simulink model "BLDC_Motor_FOC_rev6"  (R2017b)
settings: Solver=FixedStepDiscrete  StartTime=0.0  StopTime=2  MaxStep=1e-4  RelTol=1e-4
libraries: powerlib x11, powerlib_meascontrol x1
settings Model: Creator=Nick  LastModifiedBy=Nick
settings CodeAppCC: StateflowObjectComments=on

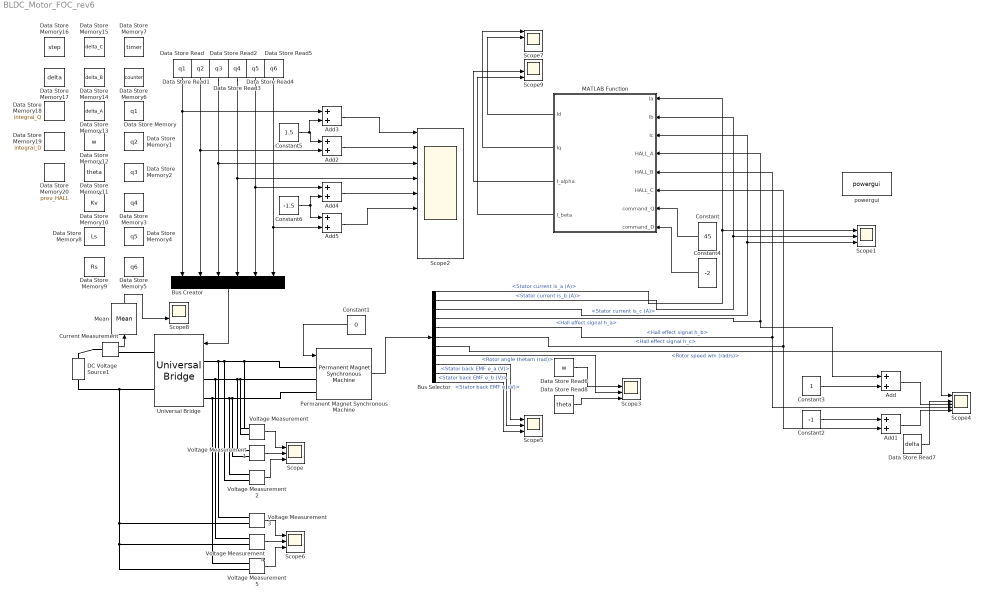
== system BLDC_Motor_FOC_rev6 ==
  Add{,1..5} (6 alike) : Sum
  Bus Creator : BusCreator  Inputs=6
  Bus Selector : BusSelector  OutputSignals=Stator current is_a (A),Stator current is_b (A),Stator current is_c (A),Hall effect signal h_a,Hall effect signal h_b,Hall effect signal h_c,Rotor speed wm (rad/s),Rotor angle thetam (rad),Stator back EMF e_a (V),Stator back EMF e_b (V),Stator back EMF e_cV)
  Constant : Constant  Value=45
  Constant1 : Constant  Value=0
  Constant2 : Constant  Value=-1
  Constant3 : Constant
  Constant4 : Constant  Value=-2
  Constant5 : Constant  Value=1.5
  Constant6 : Constant  Value=-1.5
  Current Measurement : powerlib/Measurements/Current Measurement  PhasorSimulation=off  OutputType=Complex  PSBequivalent=0
  DC Voltage Source1 : powerlib/Electrical Sources/DC Voltage Source  Amplitude=48  Measurements=None
  Data Store Memory : DataStoreMemory  DataStoreName=q1  ReadBeforeWriteMsg=warning  WriteAfterWriteMsg=warning  WriteAfterReadMsg=warning  ShowAdditionalParam=off  OutDataTypeStr=double
  Data Store Memory1 : DataStoreMemory  DataStoreName=q2  ReadBeforeWriteMsg=warning  WriteAfterWriteMsg=warning  WriteAfterReadMsg=warning  ShowAdditionalParam=off  OutDataTypeStr=double
  Data Store Memory10 : DataStoreMemory  DataStoreName=Kv  ReadBeforeWriteMsg=warning  WriteAfterWriteMsg=warning  WriteAfterReadMsg=warning  InitialValue=100  ShowAdditionalParam=off  OutDataTypeStr=double
  Data Store Memory11 : DataStoreMemory  DataStoreName=theta  ReadBeforeWriteMsg=warning  WriteAfterWriteMsg=warning  WriteAfterReadMsg=warning  ShowAdditionalParam=off  OutDataTypeStr=double
  Data Store Memory12 : DataStoreMemory  DataStoreName=w  ReadBeforeWriteMsg=warning  WriteAfterWriteMsg=warning  WriteAfterReadMsg=warning  ShowAdditionalParam=off  OutDataTypeStr=double
  Data Store Memory13 : DataStoreMemory  DataStoreName=delta_A  ReadBeforeWriteMsg=warning  WriteAfterWriteMsg=warning  WriteAfterReadMsg=warning  ShowAdditionalParam=off  OutDataTypeStr=double
  Data Store Memory14 : DataStoreMemory  DataStoreName=delta_B  ReadBeforeWriteMsg=warning  WriteAfterWriteMsg=warning  WriteAfterReadMsg=warning  ShowAdditionalParam=off  OutDataTypeStr=double
  Data Store Memory15 : DataStoreMemory  DataStoreName=delta_C  ReadBeforeWriteMsg=warning  WriteAfterWriteMsg=warning  WriteAfterReadMsg=warning  ShowAdditionalParam=off  OutDataTypeStr=double
  Data Store Memory16 : DataStoreMemory  DataStoreName=step  ReadBeforeWriteMsg=warning  WriteAfterWriteMsg=warning  WriteAfterReadMsg=warning  InitialValue=5e-6  ShowAdditionalParam=off  OutDataTypeStr=double
  Data Store Memory17 : DataStoreMemory  DataStoreName=delta  ReadBeforeWriteMsg=warning  WriteAfterWriteMsg=warning  WriteAfterReadMsg=warning  ShowAdditionalParam=off  OutDataTypeStr=double
  Data Store Memory18 : DataStoreMemory  DataStoreName=integral_Q  ReadBeforeWriteMsg=warning  WriteAfterWriteMsg=warning  WriteAfterReadMsg=warning  ShowAdditionalParam=off  OutDataTypeStr=double
  Data Store Memory19 : DataStoreMemory  DataStoreName=integral_D  ReadBeforeWriteMsg=warning  WriteAfterWriteMsg=warning  WriteAfterReadMsg=warning  ShowAdditionalParam=off  OutDataTypeStr=double
  Data Store Memory2 : DataStoreMemory  DataStoreName=q3  ReadBeforeWriteMsg=warning  WriteAfterWriteMsg=warning  WriteAfterReadMsg=warning  ShowAdditionalParam=off  OutDataTypeStr=double
  Data Store Memory20 : DataStoreMemory  DataStoreName=prev_HALL  ReadBeforeWriteMsg=warning  WriteAfterWriteMsg=warning  WriteAfterReadMsg=warning  ShowAdditionalParam=off  OutDataTypeStr=double
  Data Store Memory3 : DataStoreMemory  DataStoreName=q4  ReadBeforeWriteMsg=warning  WriteAfterWriteMsg=warning  WriteAfterReadMsg=warning  ShowAdditionalParam=off  OutDataTypeStr=double
  Data Store Memory4 : DataStoreMemory  DataStoreName=q5  ReadBeforeWriteMsg=warning  WriteAfterWriteMsg=warning  WriteAfterReadMsg=warning  ShowAdditionalParam=off  OutDataTypeStr=double
  Data Store Memory5 : DataStoreMemory  DataStoreName=q6  ReadBeforeWriteMsg=warning  WriteAfterWriteMsg=warning  WriteAfterReadMsg=warning  ShowAdditionalParam=off  OutDataTypeStr=double
  Data Store Memory6 : DataStoreMemory  DataStoreName=counter  ReadBeforeWriteMsg=warning  WriteAfterWriteMsg=warning  WriteAfterReadMsg=warning  ShowAdditionalParam=off  OutDataTypeStr=double
  Data Store Memory7 : DataStoreMemory  DataStoreName=timer  ReadBeforeWriteMsg=warning  WriteAfterWriteMsg=warning  WriteAfterReadMsg=warning  ShowAdditionalParam=off  OutDataTypeStr=double
  Data Store Memory8 : DataStoreMemory  DataStoreName=Ls  ReadBeforeWriteMsg=warning  WriteAfterWriteMsg=warning  WriteAfterReadMsg=warning  InitialValue=.0085  ShowAdditionalParam=off  OutDataTypeStr=double
  Data Store Memory9 : DataStoreMemory  DataStoreName=Rs  ReadBeforeWriteMsg=warning  WriteAfterWriteMsg=warning  WriteAfterReadMsg=warning  InitialValue=.0485  ShowAdditionalParam=off  OutDataTypeStr=double
  Data Store Read : DataStoreRead  DataStoreName=q1
  Data Store Read1 : DataStoreRead  DataStoreName=q2
  Data Store Read2 : DataStoreRead  DataStoreName=q3
  Data Store Read3 : DataStoreRead  DataStoreName=q4
  Data Store Read4 : DataStoreRead  DataStoreName=q5
  Data Store Read5 : DataStoreRead  DataStoreName=q6
  Data Store Read6 : DataStoreRead  DataStoreName=w
  Data Store Read7 : DataStoreRead  DataStoreName=delta
  Data Store Read8 : DataStoreRead  DataStoreName=theta
  MATLAB Function : MATLAB Function  TreatAsAtomicUnit=on
  Mean : powerlib_meascontrol/Measurements/Mean  Freq=60  Vinit=0  Ts=5e-05
  Permanent Magnet Synchronous Machine : powerlib/Machines/Permanent Magnet Synchronous Machine  NbPhases=3  FluxDistribution=Trapezoidal  RotorType=Round  MechanicalLoad=Torque Tm  PresetModel=No  ShowDetailedParameters=on  MeasurementBus=off  Resistance=0.0485  Inductance=8.5e-3  dqInductances=[8.5e-3,8.5e-3]  La=0.000395  MachineConstant=Voltage Constant (V_peak L-L / krpm)  Flux=0.1194  VoltageCst=100.0283  TorqueCst=0.9552  Flat=120  Mechanical=[0.0027 0.0004924 4 0]  PolePairs=4  InitialConditions=[0,0, 0,0]  InitialConditions5ph=[0 0 0 0 0 0]  TsPowergui=0  TsBlock=-1  RefAngle=Aligned with phase A axis (original Park)
      settings: SourceProductName=Simscape Power Systems
  Scope{,1,5..6,8} (5 alike) : Scope  NumInputPorts=3
  Scope2 : Scope  NumInputPorts=9
  Scope3 : Scope  NumInputPorts=4
  Scope4 : Scope  NumInputPorts=6
  Scope7 : Scope  NumInputPorts=4
  Scope9 : Scope  NumInputPorts=6
  Universal Bridge : powerlib/Power Electronics/Universal Bridge  Arms=3  SnubberResistance=1e5  SnubberCapacitance=inf  Device=MOSFET / Diodes  Ron=1e-3  Lon=0  ForwardVoltages="[  0  0  ]"  ForwardVoltage=0  GTOparameters=[ 10e-6 , 20e-6 ]  IGBTparameters=[ 1e-6 , 2e-6 ]  Measurements=None  Measurements_2=None  converterType=Rectifier
  Voltage Measurement{,1..5} (6 alike) : powerlib/Measurements/Voltage Measurement  PhasorSimulation=off  OutputType=Complex  PSBequivalent=0
  powergui : powerlib/powergui  Priority=1  SimulationMode=Discrete  SampleTime=5e-5  frequency=60  Iterations=50  frequencyindice=0  Pbase=100e6  ErrMax=1e-4  UnitsV=kV  UnitsW=MW  buscounter=0  FunctionMessages=off  echomessages=off  EnableUseOfTLC=off  CurrentSourceSwitches=off  DisableSnubberDevices=off  DisableRonSwitches=off  DisableVfSwitches=off  DisplayEquations=off  SolverType=Tustin/Backward Euler (TBE)  Interpol=off  ExternalGateDelay=off  methode=off  Ts=100  x0status=blocks  SPID=off  SwTol=0  HookPort=off  RestoreLinks=warning  ResistiveCurrentMeasurement=off  Frange=[0:2:500]  Ylog=off  Xlog=on  ShowGrid=off  save=off  variable=ZData  structure=0  ZoomFFT=off  StartTime=0.0  cycles=1  DisplayStyle=1  fundamental=60  FreqAxis=off  MaxFrequency=1000  frequencyindicesteady=1  RmsSteady=1  display=off
  wires:
  Permanent Magnet Synchronous Machine/1 -> Bus Selector/1
  Bus Selector/1 -> MATLAB Function/1(Ia), Scope1/1  "<Stator current is_a (A)>"
  Constant/1 -> MATLAB Function/7(command_Q)
  Bus Selector/5 -> Scope4/5, MATLAB Function/5(HALL_B)  "<Hall effect signal h_b>"
  Bus Selector/6 -> Add1/2, MATLAB Function/6(HALL_C)  "<Hall effect signal h_c>"
  Bus Selector/4 -> Add/1, MATLAB Function/4(HALL_A)  "<Hall effect signal h_a>"
  Voltage Measurement/1 -> Scope/1
  Bus Creator/1 -> Universal Bridge/1
  Constant3/1 -> Add/2
  Constant2/1 -> Add1/1
  Add1/1 -> Scope4/6
  Add/1 -> Scope4/4
  Data Store Read/1 -> Add3/1, Bus Creator/1
  Data Store Read2/1 -> Scope2/3, Bus Creator/3
  Data Store Read3/1 -> Scope2/4, Bus Creator/4
  Data Store Read4/1 -> Add4/1, Bus Creator/5
  Constant1/1 -> Permanent Magnet Synchronous Machine/1
  Bus Selector/7 -> Scope4/1  "<Rotor speed wm (rad/s)>"
  Voltage Measurement4/1 -> Scope6/2
  Voltage Measurement5/1 -> Scope6/3
  Data Store Read1/1 -> Add2/2, Bus Creator/2
  Bus Selector/8 -> Scope3/3  "<Rotor angle thetam (rad)>"
  Add2/1 -> Scope2/2
  Constant5/1 -> Add3/2, Add2/1
  Add4/1 -> Scope2/5
  Add5/1 -> Scope2/6
  Constant6/1 -> Add5/1, Add4/2
  Data Store Read5/1 -> Add5/2, Bus Creator/6
  Bus Selector/9 -> Scope5/1  "<Stator back EMF e_a (V)>"
  Bus Selector/10 -> Scope5/2  "<Stator back EMF e_b (V)>"
  Bus Selector/11 -> Scope5/3  "<Stator back EMF e_cV)>"
  Add3/1 -> Scope2/1
  Voltage Measurement3/1 -> Scope6/1
  Bus Selector/2 -> MATLAB Function/2(Ib), Scope1/2  "<Stator current is_b (A)>"
  Bus Selector/3 -> MATLAB Function/3(Ic), Scope1/3  "<Stator current is_c (A)>"
  Voltage Measurement1/1 -> Scope/2
  Voltage Measurement2/1 -> Scope/3
  Data Store Read6/1 -> Scope3/2
  Data Store Read7/1 -> Scope4/3
  MATLAB Function/1(Id) -> Scope7/2
  MATLAB Function/2(Iq) -> Scope7/1
  Data Store Read8/1 -> Scope3/4
  Constant4/1 -> MATLAB Function/8(command_D)
  Current Measurement/1 -> Mean/1
  Mean/1 -> Scope8/3
  MATLAB Function/3(I_alpha) -> Scope9/4
  MATLAB Function/4(I_beta) -> Scope9/6
  connections:
  Universal Bridge/LConn1 -- Voltage Measurement3/LConn1 -- Voltage Measurement2/LConn2 -- Voltage Measurement/LConn1 -- Permanent Magnet Synchronous Machine/LConn1
  Universal Bridge/LConn2 -- Voltage Measurement4/LConn1 -- Voltage Measurement1/LConn1 -- Permanent Magnet Synchronous Machine/LConn2 -- Voltage Measurement/LConn2
  Universal Bridge/LConn3 -- Voltage Measurement5/LConn1 -- Voltage Measurement2/LConn1 -- Permanent Magnet Synchronous Machine/LConn3 -- Voltage Measurement1/LConn2
  Universal Bridge/RConn2 -- Voltage Measurement3/LConn2 -- Voltage Measurement4/LConn2 -- Voltage Measurement5/LConn2 -- DC Voltage Source1/LConn1
  Universal Bridge/RConn1 -- Current Measurement/RConn1
  Current Measurement/LConn1 -- DC Voltage Source1/RConn1

== matlab function BLDC_Motor_FOC_rev6/MATLAB Function ==
  settings: updateMethod=DISCRETE  sampleTime=50e-7  description=Direct Current calculated from the parke transformation
  data Id settings: description=Direct Current calcultated from parke transformation
  data Iq settings: description=Quadrature Current calcultated from parke transformation
  data Ia settings: description=Phase A Armature current from motor
  data Ib settings: description=Phase B Armature current from motor
  data Ic settings: description=Phase C Armature current from motor
  data HALL_A settings: description=Input from hall affect sensor Phase A
  data HALL_B settings: description=Input from hall affect sensor Phase B
  data HALL_C settings: description=Input from hall affect sensor Phase C
  data command_Q settings: description=Input command from user, a percentage of 0 to 30 amps.
  data q1 settings: description=Gate of q1 (Top FET of Phase A)
  data q2 settings: description=Gate of q2 (Bottom FET of Phase A)
  data q3 settings: description=Gate of q3 (Top FET of Phase B)
  data q4 settings: description=Gate of q4 (Bottom FET of Phase B)
  data q5 settings: description=Gate of q5 (Top FET of Phase C)
  data q6 settings: description=Gate of q6 (Bottom FET of Phase C)
  data counter settings: description=Counter variable used to help set PWM in Trapezoid control mode
  data timer settings: description=Keeps a running time of the program
  data I_alpha settings: description=Corrected Phase A current after PI controller and Parke/Clarke transforms
  data I_beta settings: description=Corrected Phase B current after PI controller and Parke/Clarke transforms
  data theta settings: description=Position of the motor calcultated using time and HALL effect sensors
  data Kv settings: description=Unused variable at the moment
  data w settings: description=Speed of the motor calcultated using time and HALL effect sensors
  data delta_A settings: description=Value of HALL effect sensor A from previous step
  data delta_B settings: description=Value of HALL effect sensor B from previous step
  data delta_C settings: description=Value of HALL effect sensor C from previous step
  data step settings: description=Length of individual time step
  data delta settings: description=Holds the time since the last HALL effect sensor changed
  data integral_Q settings: description=Running value of the integral of the Quadrature current by the PI controller
  data integral_D settings: description=Running value of the integral of the Direct current by the PI controller
  data prev_HALL settings: description=Describes which HALL effect sensor was the last to change to determine the direction of the motor
  data: Id output; Iq output; Ia input size=1; Ib input size=1; Ic input size=1; HALL_A input; HALL_B input; HALL_C input size=1; command_Q input size=1; q1 data_store_memory; q2 data_store_memory; q3 data_store_memory; q4 data_store_memory; q5 data_store_memory; q6 data_store_memory; counter data_store_memory; timer data_store_memory; I_alpha output; I_beta output; theta data_store_memory; Kv data_store_memory; w data_store_memory; delta_A data_store_memory; delta_B data_store_memory; delta_C data_store_memory; step data_store_memory; delta data_store_memory; integral_Q data_store_memory; integral_D data_store_memory; prev_HALL data_store_memory; command_D input
function [Id,Iq,I_alpha, I_beta] = control(Ia,Ib,Ic,HALL_A,HALL_B,HALL_C,command_Q,command_D)

% most of the global variables that are used throughout the program are
% created and listed here
global counter     % Counter for duty cycle
global delta       % Time since previous HALL sensor
global step        % Sample period
global delta_A     % Value of HALL A one step prior
global delta_B     % Value of HALL B one step prior
global delta_C     % Value of HALL C one step prior
global w           % Speed in radians per second
global theta       % Angle in radians
global timer       % Time since start of program
global integral_Q  % Value of descrete integral for Q current
global integral_D  % Value of descrete integral for D current

A = 0; % Sets initial value for phase A voltage
B = 0; % Sets initial value for phase B voltage
C = 0; % Sets initial value for phase C voltage

% Using current readings from the current sensors we calculate the alpha
% and beta currents of the motor
[I_alpha,I_beta] = clarke(Ia,Ib,Ic);

% Continuously tracking the amount of time since the previous Hall effecto
% sensor reading to keep track of speed and position of motor
delta = delta + step; 

% Continuously keeps track of the time passed since the beginning of the
% program to change when we switch from trapezpoidal to FOC
timer = timer + step; 

if timer >= 0.0001 % Problem in function fix later
    read_pos(HALL_A,HALL_B,HALL_C); % Keeps track of the position of the motor
end


delta_A = HALL_A; % Saves previous state of Hall effect sensor A
delta_B = HALL_B; % Saves previous state of Hall effect sensor B
delta_C = HALL_C; % Saves previous state of Hall effect sensor C

theta = theta + w*step; % Integrating to keep track of angle

[Id,Iq] = park(I_alpha,I_beta,4*theta); % Calculate direct and quadrature currents

counter = counter + 1; % Keeping track of duty cycle

% Runs trapezoidal control for .1 seconds then flips to FOC
if timer < .1
    trapezoid(command_Q,HALL_A,HALL_B,HALL_C);

% Flipping Field Oriented Control
else
    % PI control for quadrature current
    error_Q = ((command_Q/100)*30) - Iq;
    integral_Q = integral_Q + (error_Q*step);
    u_Q = 1000*integral_Q + 1000*error_Q;
    
    % PI control for direct current
    error_D = (command_D - Id);
    integral_D = integral_D + (error_D*step);
    u_D = 1000*integral_D + 1000*error_D;
    
    % Calculate inverse parke transformation for PI control output
    [I_alpha,I_beta] = inverse_parke(u_D,u_Q,4*theta);
    
    % Calculate inverse clarke transformation for PI control output
    [A,B,C] = inverse_clarke(I_alpha,I_beta);
    % Raises or lowers voltages based on coontrol signal
    regulate(A,B,C,Ia,Ib,Ic); 
end
    
end

% regulate is a function that comapares the values of the 
% voltages on the line and tries to raise them if they are below
% the value that the PI controller is asking for
% or lowers them if the actual value is less than what the PI controller
% asks for
function regulate(command_A,command_B,command_C,A,B,C)
    global q1
    global q2
    global q3
    global q4
    global q5
    global q6
    
    if A < command_A
        q1 = 1;
        q2 = 0;
    else
        q1 = 0;
        q2 = 1;
    end
    if B < command_B
        q3 = 1;
        q4 = 0;
    else
        q3 = 0;
        q4 = 1;
    end
    if C < command_C
        q5 = 1;
        q6 = 0;
    else
        q5 = 0;
        q6 = 1;
    end
end


% This function takes in alpha/beta voltages/currents and the angle of the
% motor computes the direct/quadrature voltages/currents
function [d,q] = park(alpha,beta,theta)
    d = cos(theta)*alpha + sin(theta)*beta;
    q = cos(theta)*beta - sin(theta)*alpha;
end

% This function takes in a/b/c voltages/currents
% and computes the alpha/beta voltages/currents
function [alpha,beta] = clarke(a,b,c)
    alpha = a;
    beta = (1/(sqrt(3))*(b-c));
end

% This function takes in direct/gaudrature voltages/currents
% and the angle of the motor and performs the reverse parke transformation
% giving alpha/beta voltages/currents
function [alpha,beta] = inverse_parke(d,q,theta)
    alpha = d*cos(theta) - q*sin(theta);
    beta = q*cos(theta) + d*sin(theta);
end


% This function takes in alpha/beta voltages/currents and 
% performs the reverse clarke transformation and returns a/b/c
% voltages/currents
function [a,b,c] = inverse_clarke(alpha,beta)
    a = alpha;
    b = (1/2)*((-alpha) + (sqrt(3)*beta));
    c = (1/2)*((-alpha) - (sqrt(3)*beta));
end

% This function takes in a counter which helps define a duty cycle
% along with a command 0 to 100 percent and the position of the motor
% via the hall affect sensors and produces a trapazoid output signal
% to the 3 half bridges
function trapezoid(command,HALL_A,HALL_B,HALL_C)
    global q1
    global q2
    global q3
    global q4
    global q5
    global q6
    global counter
    if counter <= command
        if HALL_A && ~HALL_B && HALL_C
            q1 = 1;
            q2 = 0;
            q3 = 0;
            q4 = 1;
            q5 = 1;
            q6 = 0;

        elseif HALL_A && ~HALL_B && ~HALL_C
            q1 = 1;
            q2 = 0;
            q3 = 0;
            q4 = 1;
            q5 = 0;
            q6 = 1;

        elseif HALL_A && HALL_B && ~HALL_C
            q1 = 1;
            q2 = 0;
            q3 = 1;
            q4 = 0;
            q5 = 0;
            q6 = 1;

        elseif ~HALL_A && HALL_B && ~HALL_C
            q1 = 0;
            q2 = 1;
            q3 = 1;
            q4 = 0;
            q5 = 0;
            q6 = 1;

        elseif ~HALL_A && HALL_B && HALL_C
            q1 = 0;
            q2 = 1;
            q3 = 1;
            q4 = 0;
            q5 = 1;
            q6 = 0; 

        elseif ~HALL_A && ~HALL_B && HALL_C
            q1 = 0;
            q2 = 1;
            q3 = 0;
            q4 = 1;
            q5 = 1;
            q6 = 0;
        end
    else
        q1 = 0;
        q2 = 0;
        q3 = 0;
        q4 = 0;
        q5 = 0;
        q6 = 0;
    end
    if counter >= 100
        counter = 0;
    end
end

% This function takes the three Hall effect sensor outputs
% along with the amount of time that has passed and integrates to keep
% track of the position of the motor for use in the parke transformations
% and inverse parke transformation
function read_pos(HALL_A,HALL_B,HALL_C)
    global prev_HALL
    global delta_A
    global delta_B
    global delta_C
    global delta 
    global w
    
    if((HALL_A-delta_A ~= 0 || HALL_B-delta_B ~= 0 || HALL_C-delta_C ~= 0))

        if HALL_A-delta_A == -1
            if prev_HALL == 3
                w = -1*((2*pi)/24)/delta;

            elseif prev_HALL == 2
                w = ((2*pi)/24)/delta;
            else
                w = 0;

            end
            prev_HALL = 1;

        elseif HALL_A-delta_A == 1
            if prev_HALL == 3
                w = -1*((2*pi)/24)/delta;

            elseif prev_HALL == 2
                w = ((2*pi)/24)/delta;
            else
                w = 0;

            end
            prev_HALL = 1;

        elseif HALL_B-delta_B == -1
            if prev_HALL == 1
                w = -1*((2*pi)/24)/delta;

            elseif prev_HALL == 3
                w = ((2*pi)/24)/delta;

            else
                w = 0;

            end
            prev_HALL = 2;

        elseif HALL_B-delta_B == 1
            if prev_HALL == 1
                w = -1*((2*pi)/24)/delta;

            elseif prev_HALL == 3
                w = ((2*pi)/24)/delta;

            else
                w = 0;

            end
            prev_HALL = 2;

        elseif HALL_C-delta_C == -1
            if prev_HALL == 2
                w = -1*((2*pi)/24)/delta;

            elseif prev_HALL == 1
                w = ((2*pi)/24)/delta;

            else
                w = 0;

            end
            prev_HALL = 3;

        elseif HALL_C-delta_C == 1
            if prev_HALL == 1
                w = ((2*pi)/24)/delta;

            elseif prev_HALL == 2
                w = -1*((2*pi)/24)/delta;

            else
                w = 0;

            end
            prev_HALL = 3;

        end

        delta = 0;
    end
end


% This function is incomplete
% it will be used as a PI controller in software
function [U] = PID(Kp,Ki,Kd)
    error = target - value;
    I = i + error*step;
end
